simulink model "loopback_task"  (Simulink 3.0)
libraries: mathlib x19, logiclib x4, stringlib x4, analoglib x2, genlib x1

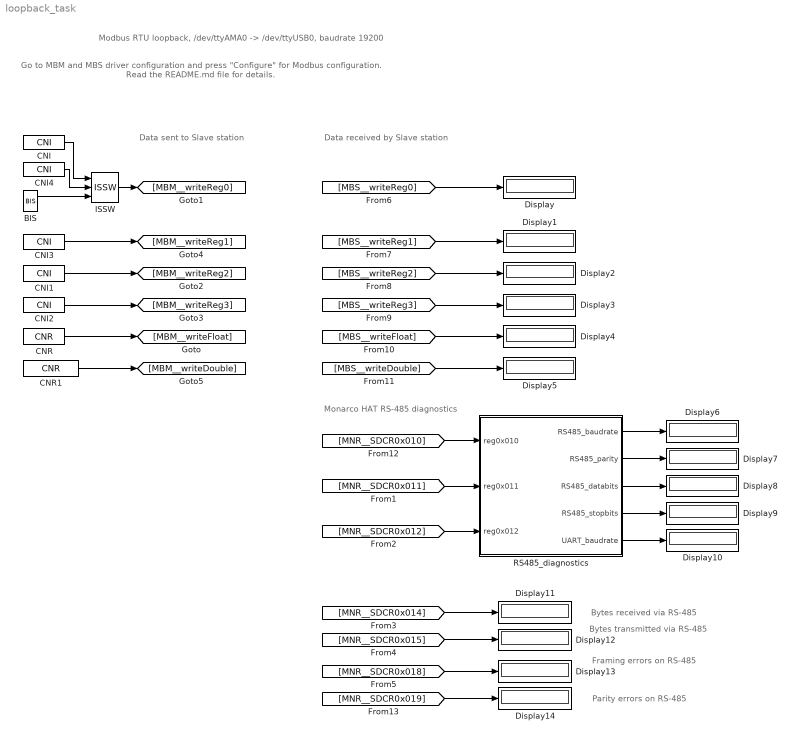
== system loopback_task ==
  note: Go to MBM and MBS driver configuration and press "Configure" for Modbus configuration.
      |
      | Read the README.md file for details.
  note: Data sent to Slave station
  note: Data received by Slave station
  note: Modbus RTU loopback, /dev/ttyAMA0 -> /dev/ttyUSB0, baudrate 19200
  note: Monarco HAT RS-485 diagnostics
  note: Bytes received via RS-485
  note: Bytes transmitted via RS-485
  note: Framing errors on RS-485
  note: Parity errors on RS-485
  BIS : genlib/BIS  Y0=off  t1=1  t2=2  t3=3  t4=4  t5=5  t6=6  t7=7  t8=8  RPT=on
  CNI : mathlib/CNI  icn=111
  CNI1 : mathlib/CNI  icn=64917
  CNI2 : mathlib/CNI  icn=-29999
  CNI3 : mathlib/CNI  icn=-95
  CNI4 : mathlib/CNI  icn=222
  CNR : mathlib/CNR  ycn=-78.57
  CNR1 : mathlib/CNR  ycn=-79315.18
  Display{,1..14} (15 alike) : Display
      Display settings: Format=Best fit
      Display1 settings: Format=Best fit
      Display10 settings: Format=Best fit
      Display11 settings: Format=Best fit
      Display12 settings: Format=Best fit
      Display13 settings: Format=Best fit
      Display14 settings: Format=Best fit
      Display2 settings: Format=Best fit
      Display3 settings: Format=Best fit
      Display4 settings: Format=short
      Display5 settings: Format=short
      Display6 settings: Format=Best fit
      Display7 settings: Format=Best fit
      Display8 settings: Format=Best fit
      Display9 settings: Format=Best fit
  ISSW : logiclib/ISSW
  RS485_diagnostics : Subsystem
      mask Type: REX sequence
  wires:
  BIS/1 -> ISSW/3
  CNI/1 -> ISSW/1
  CNI1/1 -> [MBM__writeReg2]
  CNI2/1 -> [MBM__writeReg3]
  CNI3/1 -> [MBM__writeReg1]
  CNI4/1 -> ISSW/2
  CNR/1 -> [MBM__writeFloat]
  CNR1/1 -> [MBM__writeDouble]
  [MNR__SDCR0x011] -> RS485_diagnostics/2(reg0x011)
  [MBS__writeFloat] -> Display4/1
  [MBS__writeDouble] -> Display5/1
  [MNR__SDCR0x010] -> RS485_diagnostics/1(reg0x010)
  [MNR__SDCR0x019] -> Display14/1
  [MNR__SDCR0x012] -> RS485_diagnostics/3(reg0x012)
  [MNR__SDCR0x014] -> Display11/1
  [MNR__SDCR0x015] -> Display12/1
  [MNR__SDCR0x018] -> Display13/1
  [MBS__writeReg0] -> Display/1
  [MBS__writeReg1] -> Display1/1
  [MBS__writeReg2] -> Display2/1
  [MBS__writeReg3] -> Display3/1
  ISSW/1 -> [MBM__writeReg0]
  RS485_diagnostics/1(RS485_baudrate) -> Display6/1
  RS485_diagnostics/2(RS485_parity) -> Display7/1
  RS485_diagnostics/3(RS485_databits) -> Display8/1
  RS485_diagnostics/4(RS485_stopbits) -> Display9/1
  RS485_diagnostics/5(UART_baudrate) -> Display10/1

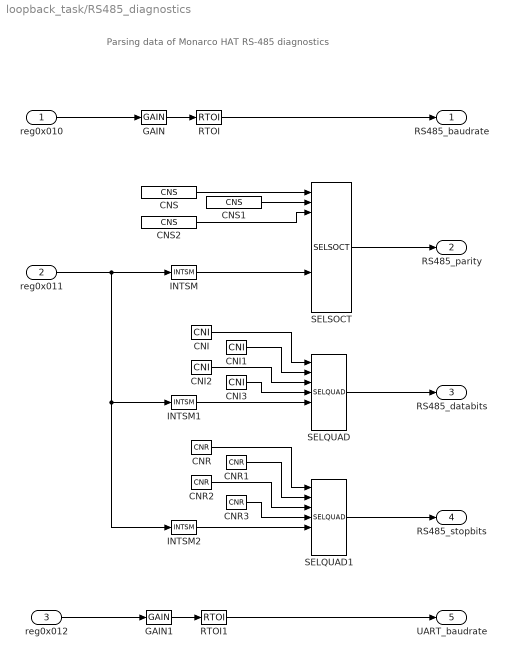
== system loopback_task/RS485_diagnostics ==
  note: Parsing data of Monarco HAT RS-485 diagnostics
  reg0x010 : Inport  Port=1
  reg0x011 : Inport  Port=2
  reg0x012 : Inport  Port=3
  CNI : mathlib/CNI  icn=5
  CNI1 : mathlib/CNI  icn=6
  CNI2 : mathlib/CNI  icn=7
  CNI3 : mathlib/CNI  icn=8
  CNR : mathlib/CNR  ycn=0.5
  CNR1 : mathlib/CNR  ycn=1.0
  CNR2 : mathlib/CNR  ycn=1.5
  CNR3 : mathlib/CNR  ycn=2.0
  CNS : stringlib/CNS  scv=0: none  nmax=0
  CNS1 : stringlib/CNS  scv=1: even  nmax=0
  CNS2 : stringlib/CNS  scv=2: odd  nmax=0
  GAIN : mathlib/GAIN  k=100
  GAIN1 : mathlib/GAIN  k=100
  INTSM : logiclib/INTSM  shift=0  mask=0x07
  INTSM1 : logiclib/INTSM  shift=3  mask=0x03
  INTSM2 : logiclib/INTSM  shift=5  mask=0x03
  RTOI : mathlib/RTOI
  RTOI1 : mathlib/RTOI
  SELQUAD : analoglib/SELQUAD  BINF=off
  SELQUAD1 : analoglib/SELQUAD  BINF=off
  SELSOCT : stringlib/SELSOCT  BINF=off  nmax=0
  RS485_baudrate : Outport  Port=1
  RS485_parity : Outport  Port=2
  RS485_databits : Outport  Port=3
  RS485_stopbits : Outport  Port=4
  UART_baudrate : Outport  Port=5
  wires:
  CNI/1 -> SELQUAD/1
  CNI1/1 -> SELQUAD/2
  CNI2/1 -> SELQUAD/3
  CNI3/1 -> SELQUAD/4
  CNR/1 -> SELQUAD1/1
  CNR1/1 -> SELQUAD1/2
  CNR2/1 -> SELQUAD1/3
  CNR3/1 -> SELQUAD1/4
  CNS/1 -> SELSOCT/1
  CNS1/1 -> SELSOCT/2
  CNS2/1 -> SELSOCT/3
  GAIN/1 -> RTOI/1
  GAIN1/1 -> RTOI1/1
  INTSM/1 -> SELSOCT/9
  INTSM1/1 -> SELQUAD/5
  INTSM2/1 -> SELQUAD1/5
  RTOI/1 -> RS485_baudrate/1
  RTOI1/1 -> UART_baudrate/1
  SELQUAD/1 -> RS485_databits/1
  SELQUAD1/1 -> RS485_stopbits/1
  SELSOCT/1 -> RS485_parity/1
  reg0x010/1 -> GAIN/1
  reg0x011/1 -> INTSM/1, INTSM1/1, INTSM2/1
  reg0x012/1 -> GAIN1/1
